simulink model "AbsVsImpl_Temporal_Logic"  (R2025b)
settings: Solver=FixedStepDiscrete  StartTime=0.0  StopTime=10.0  FixedStep=0.01  RelTol=1e-3
settings Model: Creator=soura  LastModifiedBy=soura

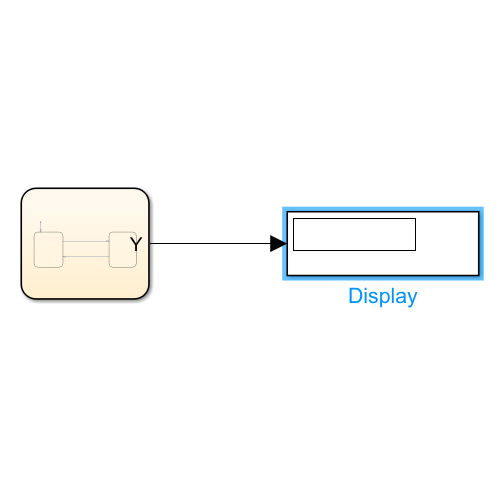
[thumbnail: Simulink's stored preview of the top-level diagram]
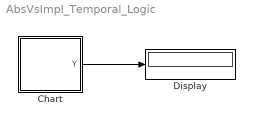
== system AbsVsImpl_Temporal_Logic ==
  Chart : Stateflow chart  TreatAsAtomicUnit=on
  Display : Display
  wires:
  Chart/1(Y) -> Display/1

== stateflow chart AbsVsImpl_Temporal_Logic/Chart ==
  state Off
    en:
    Y=0;
  state On
    en:
    Y=1;
  (default) -> Off
  Off -> On : after(20,msec)
  On -> Off : after(5,tick)
  data: Y output
